simulink model "PVmppt"  (R2018b)
settings: Solver=FixedStepAuto  StartTime=0.0  StopTime=Inf  FixedStep=T  RelTol=1e-3
PostLoadFcn:
  | , if any(exist('dsrtsu_mdlpostloadfcn', 'file') ~= 0), dsrtsu_mdlpostloadfcn('Execute', bdroot); end,
InitFcn:
  | , if any(exist('dsmpb_private', 'file') ~= 0), dsmpb_private('dsmpb_mdlclblib', 'Init', bdroot); end,
values from neighbouring files (symbols this model uses):
  fixedgain_i1 = 10*1000/(3*100)    (= 33.3333333333)    [param.m]
  fixedgain_v3 = 10*22000/(3*100*2.5)    (= 293.333333333)    [param.m]
  fixedgain_v4 = 10*22000/(3*100*2.5)    (= 293.333333333)    [param.m]
  gain_i1 = 1    [param.m]
  gain_v1 = 1    [param.m]
  gain_v3 = 1    [param.m]
  gain_v4 = 1    [param.m]
  offset_i1 = 0.25    [param.m]
  offset_v1 = 0.15    [param.m]
  offset_v3 = 0.6    [param.m]
  offset_v4 = 0.2    [param.m]
undefined symbols (not defined in the file or in its folder): fixedgain_vc1
libraries: rti1202lib_adc_class1 x4, rtiproclib x3
PreSaveFcn:
  | , if any(exist('dsmpb_private', 'file') ~= 0), dsmpb_private('dsmpb_mdlclblib', 'PreSave', bdroot); end,
CloseFcn:
  | , if any(exist('dsmpb_private', 'file') ~= 0), dsmpb_private('dsmpb_mdlclblib', 'Close', bdroot); end,
Description:
  | Standard RTI1202 template.
  | Supported MATLAB version:  R2018b.
settings Model: Tag=RTI1202  DSRTSU_INTERNAL_RTI_VER=550  DSRTSU_INTERNAL_RTI_TYPE=rti1202  RTICANMMDATA=struct('GeneralSetupData',struct('modelroot','C:\marcos\LSPyC_Varios\BOOST','generalsettings',struct('filesettings',struct('destfolder',struct('Name','RTICANMM_FILES','Check',1),'buildfolder',struct('Name','.','Check',1),'AbsDestfolder',struct('Name','C:\marcos\LSPyC_Varios\BOOST\RTICANMM_FILES'),'AbsBuildfolder',struct('Name','C:\marcos\LSPyC_Varios\BOOST'))),'options',struct('addpaths',1,'rmpaths',1,'addtrcexclusion',true,'cannavigator',struct('checkmonitoring',0),'show_usrtrc',0,'use_usrtrc',0),'advanced',struct('options',ones(1,100)),'MPSetup',{{}},'RTI',struct('Type','RTI1202','Ver','7.13','Date','02-Nov-2019'),'modelname','PVmppt','block','PVmppt'))  DSRTSU_INTERNAL_RTIFPGA=150  DSMPB_ID_DATA={}  Creator=Admin  LastModifiedBy=Admin
settings OptimizationCC: BlockReduction=off  OptimizeBlockIOStorage=off  BufferReuse=off  GlobalBufferReuse=off  ExpressionFolding=off  LocalBlockOutputs=off  OptimizeDataStoreBuffers=off  BusAssignmentInplaceUpdate=off
settings DebuggingCC: LibraryContextMissingDiagnostic=none
settings HardwareCC: ProdBitPerPointer=32  ProdBitPerSizeT=32  ProdBitPerPtrDiffT=32  ProdLargestAtomicInteger=Integer  ProdEndianess=BigEndian  ProdWordSize=32  ProdHWDeviceType=Custom Processor->Custom  TargetIntDivRoundTo=Zero  TargetEndianess=BigEndian  TargetHWDeviceType=Custom Processor->Custom
settings SFSimCC: SimUseLocalCustomCode=off  MATLABDynamicMemAlloc=off
settings RTWCC: SystemTargetFile=rti1202.tlc  MakeCommand=make_rti  TemplateMakefile=rti1202.tmf  Description=dSPACE DS1202 Hardware Platform  RTWUseLocalCustomCode=off
settings CodeAppCC: StateflowObjectComments=on
settings STFCustomTargetCC: ParMdlRefBuildCompliant=on  SystemTargetFile=rti1202.tlc
settings GRTTargetCC: TargetLangStandard=C89/C90 (ANSI)  CompOptLevelCompliant=off  ConcurrentExecutionCompliant=off  CombineOutputUpdateFcns=off  MatFileLogging=off  CPPClassGenCompliant=off  UseToolchainInfoCompliant=off
settings ConfigComp: CovMetricSettings=dswe

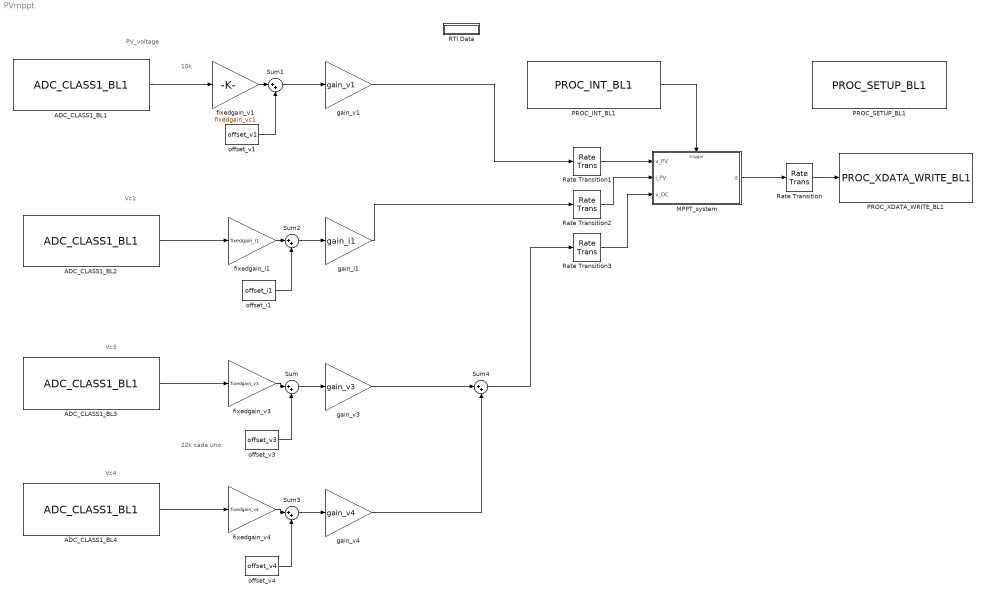
== system PVmppt ==
  note: 22k cada uno
  note: Vc3
  note: 10k
  note: Vc1
  note: PV_voltage
  note: Vc4
  ADC_CLASS1_BL1 : rti1202lib_adc_class1/ADC_CLASS1_BL1  DSProperties=struct('RTI',struct('Version',uint32(1),'BlockType',struct('isSLSource',uint8(1),'isSLSink',uint8(1),'isHWSource',uint8(0),'isHWSink',uint8(1),'isSetup',uint8(0),'isInline',uint8(1),'isNonInline',uint8(0),'isInterrupt',uint8(0),'isChannelwise',uint8(1)),'IOBoardType',{{'DS120X','STD','ADCC1'}},'UnitType','ADC','Identifier','ADC','DialogType','ML','BlockSet','NONE','SlaveProcessor','NONE'))  RTIBlockInterface=struct('InputPortsActive',0,'InputPortsWidth',int32(1),'InputPortsDataType',{{'SS_BOOLEAN'}},'InputPortsName',{{'Continue'}},'OutputPortsActive',[1 0],'OutputPortsWidth',int32([1 1]),'OutputPortsDataType',{{'SS_DOUBLE','SS_INT16'}},'OutputPortsName',{{'ADC','Status'}},'DialogFcn','rti120xstdadcc1adcgui','SampleTime',{{-1}},'InitLevel',3,'IconTransparency','on','BlockDisplay',{{['ADC CL1\nChannel: 1'],'center'}},'BlockName',struct('Token',{{'ADC_CLASS1_BL1'}}))  RTIBlockParameters=struct('ReadMode',{{1,'OFF',[1 2]}},'ChannelNo',{{1,'OFF',[]}},'ConversionMode',{{1,'OFF',[1 2]}},'TriggerSource',{{1,'OFF',[1 2]}},'TriggerLineIn',{{1,'OFF',[1 16]}},'SampleMode',{{1,'OFF',[1 2]}},'BurstTriggerSource',{{1,'OFF',[1 2]}},'BurstTriggerLine',{{1,'OFF',[1 16]}},'ConvTriggerSource',{{3,'OFF',[1 3]}},'ConvTriggerLine',{{1,'OFF',[1 16]}},'ConvPeriod',{{'100e-6','OFF',[1e-6 1.34]}},'ConvPeriodCheck',{{0,'OFF',[]}},'BurstSize',{{'10','OFF',[]}},'BurstSizeCheck',{{0,'OFF',[]}},'DataSetOffset',{{'0','OFF',[]}},'DataSetOffsetCheck',{{0,'OFF',[]}},'DataSetLength',{{'1','OFF',[]}},'DataSetLengthCheck',{{0,'OFF',[]}},'EnableTriggerEvent',{{0,'OFF',[0 1]}},'TriggerMode',{{2,'OFF',[1 3]}},'TriggerLineOut',{{1,'OFF',[1 16]}},'ADCSWStartEnable',{{0,'OFF',[0 1]}},'SampleTime',{{'-1','OFF',[-1 inf]}},'SampleTimeCheck',{{1,'OFF',[]}},'StatusPortEnable',{{0,'OFF',[0 1]}},'TLCFileName',{{'rti120xadc_c1_adc','OFF',[]}})  RTISFcnParameters=struct('ReadMode','int16','ChannelNo','int16','ConversionMode','int16','TriggerSource','int16','TriggerLineIn','int16','SampleMode','int16','BurstTriggerSource','int16','BurstTriggerLine','int16','ConvTriggerSource','int16','ConvTriggerLine','int16','ConvPeriod','double','BurstSize','int16','DataSetOffset','int16','DataSetLength','int16','EnableTriggerEvent','int16','TriggerMode','int16','TriggerLineOut','int16','ADCSWStartEnable','int16','SampleTime','double','StatusPortEnable','int16','TLCFileName','char')  RTIBlockParaDefault=struct('ReadMode',1,'ChannelNo',1,'ConversionMode',1,'TriggerSource',1,'TriggerLineIn',1,'SampleMode',1,'BurstTriggerSource',1,'BurstTriggerLine',1,'ConvTriggerSource',3,'ConvTriggerLine',1,'ConvPeriod',0.0001,'ConvPeriodCheck',0,'BurstSize',10,'BurstSizeCheck',0,'DataSetOffset',0,'DataSetOffsetCheck',0,'DataSetLength',1,'DataSetLengthCheck',0,'EnableTriggerEvent',0,'TriggerMode',2,'TriggerLineOut',1,'ADCSWStartEnable',0,'SampleTime',-1,'SampleTimeCheck',1,'StatusPortEnable',0,'TLCFileName','rti120xadc_c1_adc')
  ADC_CLASS1_BL2 : rti1202lib_adc_class1/ADC_CLASS1_BL1  DSProperties=struct('RTI',struct('Version',uint32(1),'BlockType',struct('isSLSource',uint8(1),'isSLSink',uint8(1),'isHWSource',uint8(0),'isHWSink',uint8(1),'isSetup',uint8(0),'isInline',uint8(1),'isNonInline',uint8(0),'isInterrupt',uint8(0),'isChannelwise',uint8(1)),'IOBoardType',{{'DS120X','STD','ADCC1'}},'UnitType','ADC','Identifier','ADC','DialogType','ML','BlockSet','NONE','SlaveProcessor','NONE'))  RTIBlockInterface=struct('InputPortsActive',0,'InputPortsWidth',int32(1),'InputPortsDataType',{{'SS_BOOLEAN'}},'InputPortsName',{{'Continue'}},'OutputPortsActive',[1 0],'OutputPortsWidth',int32([1 1]),'OutputPortsDataType',{{'SS_DOUBLE','SS_INT16'}},'OutputPortsName',{{'ADC','Status'}},'DialogFcn','rti120xstdadcc1adcgui','SampleTime',{{-1}},'InitLevel',3,'IconTransparency','on','BlockDisplay',{{['ADC CL1\nChannel: 9'],'center'}},'BlockName',struct('Token',{{'ADC_CLASS1_BL1'}}))  RTIBlockParameters=struct('ReadMode',{{1,'OFF',[1 2]}},'ChannelNo',{{9,'OFF',[]}},'ConversionMode',{{1,'OFF',[1 2]}},'TriggerSource',{{1,'OFF',[1 2]}},'TriggerLineIn',{{1,'OFF',[1 16]}},'SampleMode',{{1,'OFF',[1 2]}},'BurstTriggerSource',{{1,'OFF',[1 2]}},'BurstTriggerLine',{{1,'OFF',[1 16]}},'ConvTriggerSource',{{3,'OFF',[1 3]}},'ConvTriggerLine',{{1,'OFF',[1 16]}},'ConvPeriod',{{'100e-6','OFF',[1e-6 1.34]}},'ConvPeriodCheck',{{0,'OFF',[]}},'BurstSize',{{'10','OFF',[]}},'BurstSizeCheck',{{0,'OFF',[]}},'DataSetOffset',{{'0','OFF',[]}},'DataSetOffsetCheck',{{0,'OFF',[]}},'DataSetLength',{{'1','OFF',[]}},'DataSetLengthCheck',{{0,'OFF',[]}},'EnableTriggerEvent',{{0,'OFF',[0 1]}},'TriggerMode',{{2,'OFF',[1 3]}},'TriggerLineOut',{{1,'OFF',[1 16]}},'ADCSWStartEnable',{{0,'OFF',[0 1]}},'SampleTime',{{'-1','OFF',[-1 inf]}},'SampleTimeCheck',{{1,'OFF',[]}},'StatusPortEnable',{{0,'OFF',[0 1]}},'TLCFileName',{{'rti120xadc_c1_adc','OFF',[]}})  RTISFcnParameters=struct('ReadMode','int16','ChannelNo','int16','ConversionMode','int16','TriggerSource','int16','TriggerLineIn','int16','SampleMode','int16','BurstTriggerSource','int16','BurstTriggerLine','int16','ConvTriggerSource','int16','ConvTriggerLine','int16','ConvPeriod','double','BurstSize','int16','DataSetOffset','int16','DataSetLength','int16','EnableTriggerEvent','int16','TriggerMode','int16','TriggerLineOut','int16','ADCSWStartEnable','int16','SampleTime','double','StatusPortEnable','int16','TLCFileName','char')  RTIBlockParaDefault=struct('ReadMode',1,'ChannelNo',1,'ConversionMode',1,'TriggerSource',1,'TriggerLineIn',1,'SampleMode',1,'BurstTriggerSource',1,'BurstTriggerLine',1,'ConvTriggerSource',3,'ConvTriggerLine',1,'ConvPeriod',0.0001,'ConvPeriodCheck',0,'BurstSize',10,'BurstSizeCheck',0,'DataSetOffset',0,'DataSetOffsetCheck',0,'DataSetLength',1,'DataSetLengthCheck',0,'EnableTriggerEvent',0,'TriggerMode',2,'TriggerLineOut',1,'ADCSWStartEnable',0,'SampleTime',-1,'SampleTimeCheck',1,'StatusPortEnable',0,'TLCFileName','rti120xadc_c1_adc')
  ADC_CLASS1_BL3 : rti1202lib_adc_class1/ADC_CLASS1_BL1  DSProperties=struct('RTI',struct('Version',uint32(1),'BlockType',struct('isSLSource',uint8(1),'isSLSink',uint8(1),'isHWSource',uint8(0),'isHWSink',uint8(1),'isSetup',uint8(0),'isInline',uint8(1),'isNonInline',uint8(0),'isInterrupt',uint8(0),'isChannelwise',uint8(1)),'IOBoardType',{{'DS120X','STD','ADCC1'}},'UnitType','ADC','Identifier','ADC','DialogType','ML','BlockSet','NONE','SlaveProcessor','NONE'))  RTIBlockInterface=struct('InputPortsActive',0,'InputPortsWidth',int32(1),'InputPortsDataType',{{'SS_BOOLEAN'}},'InputPortsName',{{'Continue'}},'OutputPortsActive',[1 0],'OutputPortsWidth',int32([1 1]),'OutputPortsDataType',{{'SS_DOUBLE','SS_INT16'}},'OutputPortsName',{{'ADC','Status'}},'DialogFcn','rti120xstdadcc1adcgui','SampleTime',{{-1}},'InitLevel',3,'IconTransparency','on','BlockDisplay',{{['ADC CL1\nChannel: 3'],'center'}},'BlockName',struct('Token',{{'ADC_CLASS1_BL1'}}))  RTIBlockParameters=struct('ReadMode',{{1,'OFF',[1 2]}},'ChannelNo',{{3,'OFF',[]}},'ConversionMode',{{1,'OFF',[1 2]}},'TriggerSource',{{1,'OFF',[1 2]}},'TriggerLineIn',{{1,'OFF',[1 16]}},'SampleMode',{{1,'OFF',[1 2]}},'BurstTriggerSource',{{1,'OFF',[1 2]}},'BurstTriggerLine',{{1,'OFF',[1 16]}},'ConvTriggerSource',{{3,'OFF',[1 3]}},'ConvTriggerLine',{{1,'OFF',[1 16]}},'ConvPeriod',{{'100e-6','OFF',[1e-6 1.34]}},'ConvPeriodCheck',{{0,'OFF',[]}},'BurstSize',{{'10','OFF',[]}},'BurstSizeCheck',{{0,'OFF',[]}},'DataSetOffset',{{'0','OFF',[]}},'DataSetOffsetCheck',{{0,'OFF',[]}},'DataSetLength',{{'1','OFF',[]}},'DataSetLengthCheck',{{0,'OFF',[]}},'EnableTriggerEvent',{{0,'OFF',[0 1]}},'TriggerMode',{{2,'OFF',[1 3]}},'TriggerLineOut',{{1,'OFF',[1 16]}},'ADCSWStartEnable',{{0,'OFF',[0 1]}},'SampleTime',{{'-1','OFF',[-1 inf]}},'SampleTimeCheck',{{1,'OFF',[]}},'StatusPortEnable',{{0,'OFF',[0 1]}},'TLCFileName',{{'rti120xadc_c1_adc','OFF',[]}})  RTISFcnParameters=struct('ReadMode','int16','ChannelNo','int16','ConversionMode','int16','TriggerSource','int16','TriggerLineIn','int16','SampleMode','int16','BurstTriggerSource','int16','BurstTriggerLine','int16','ConvTriggerSource','int16','ConvTriggerLine','int16','ConvPeriod','double','BurstSize','int16','DataSetOffset','int16','DataSetLength','int16','EnableTriggerEvent','int16','TriggerMode','int16','TriggerLineOut','int16','ADCSWStartEnable','int16','SampleTime','double','StatusPortEnable','int16','TLCFileName','char')  RTIBlockParaDefault=struct('ReadMode',1,'ChannelNo',1,'ConversionMode',1,'TriggerSource',1,'TriggerLineIn',1,'SampleMode',1,'BurstTriggerSource',1,'BurstTriggerLine',1,'ConvTriggerSource',3,'ConvTriggerLine',1,'ConvPeriod',0.0001,'ConvPeriodCheck',0,'BurstSize',10,'BurstSizeCheck',0,'DataSetOffset',0,'DataSetOffsetCheck',0,'DataSetLength',1,'DataSetLengthCheck',0,'EnableTriggerEvent',0,'TriggerMode',2,'TriggerLineOut',1,'ADCSWStartEnable',0,'SampleTime',-1,'SampleTimeCheck',1,'StatusPortEnable',0,'TLCFileName','rti120xadc_c1_adc')
  ADC_CLASS1_BL4 : rti1202lib_adc_class1/ADC_CLASS1_BL1  DSProperties=struct('RTI',struct('Version',uint32(1),'BlockType',struct('isSLSource',uint8(1),'isSLSink',uint8(1),'isHWSource',uint8(0),'isHWSink',uint8(1),'isSetup',uint8(0),'isInline',uint8(1),'isNonInline',uint8(0),'isInterrupt',uint8(0),'isChannelwise',uint8(1)),'IOBoardType',{{'DS120X','STD','ADCC1'}},'UnitType','ADC','Identifier','ADC','DialogType','ML','BlockSet','NONE','SlaveProcessor','NONE'))  RTIBlockInterface=struct('InputPortsActive',0,'InputPortsWidth',int32(1),'InputPortsDataType',{{'SS_BOOLEAN'}},'InputPortsName',{{'Continue'}},'OutputPortsActive',[1 0],'OutputPortsWidth',int32([1 1]),'OutputPortsDataType',{{'SS_DOUBLE','SS_INT16'}},'OutputPortsName',{{'ADC','Status'}},'DialogFcn','rti120xstdadcc1adcgui','SampleTime',{{-1}},'InitLevel',3,'IconTransparency','on','BlockDisplay',{{['ADC CL1\nChannel: 4'],'center'}},'BlockName',struct('Token',{{'ADC_CLASS1_BL1'}}))  RTIBlockParameters=struct('ReadMode',{{1,'OFF',[1 2]}},'ChannelNo',{{4,'OFF',[]}},'ConversionMode',{{1,'OFF',[1 2]}},'TriggerSource',{{1,'OFF',[1 2]}},'TriggerLineIn',{{1,'OFF',[1 16]}},'SampleMode',{{1,'OFF',[1 2]}},'BurstTriggerSource',{{1,'OFF',[1 2]}},'BurstTriggerLine',{{1,'OFF',[1 16]}},'ConvTriggerSource',{{3,'OFF',[1 3]}},'ConvTriggerLine',{{1,'OFF',[1 16]}},'ConvPeriod',{{'100e-6','OFF',[1e-6 1.34]}},'ConvPeriodCheck',{{0,'OFF',[]}},'BurstSize',{{'10','OFF',[]}},'BurstSizeCheck',{{0,'OFF',[]}},'DataSetOffset',{{'0','OFF',[]}},'DataSetOffsetCheck',{{0,'OFF',[]}},'DataSetLength',{{'1','OFF',[]}},'DataSetLengthCheck',{{0,'OFF',[]}},'EnableTriggerEvent',{{0,'OFF',[0 1]}},'TriggerMode',{{2,'OFF',[1 3]}},'TriggerLineOut',{{1,'OFF',[1 16]}},'ADCSWStartEnable',{{0,'OFF',[0 1]}},'SampleTime',{{'-1','OFF',[-1 inf]}},'SampleTimeCheck',{{1,'OFF',[]}},'StatusPortEnable',{{0,'OFF',[0 1]}},'TLCFileName',{{'rti120xadc_c1_adc','OFF',[]}})  RTISFcnParameters=struct('ReadMode','int16','ChannelNo','int16','ConversionMode','int16','TriggerSource','int16','TriggerLineIn','int16','SampleMode','int16','BurstTriggerSource','int16','BurstTriggerLine','int16','ConvTriggerSource','int16','ConvTriggerLine','int16','ConvPeriod','double','BurstSize','int16','DataSetOffset','int16','DataSetLength','int16','EnableTriggerEvent','int16','TriggerMode','int16','TriggerLineOut','int16','ADCSWStartEnable','int16','SampleTime','double','StatusPortEnable','int16','TLCFileName','char')  RTIBlockParaDefault=struct('ReadMode',1,'ChannelNo',1,'ConversionMode',1,'TriggerSource',1,'TriggerLineIn',1,'SampleMode',1,'BurstTriggerSource',1,'BurstTriggerLine',1,'ConvTriggerSource',3,'ConvTriggerLine',1,'ConvPeriod',0.0001,'ConvPeriodCheck',0,'BurstSize',10,'BurstSizeCheck',0,'DataSetOffset',0,'DataSetOffsetCheck',0,'DataSetLength',1,'DataSetLengthCheck',0,'EnableTriggerEvent',0,'TriggerMode',2,'TriggerLineOut',1,'ADCSWStartEnable',0,'SampleTime',-1,'SampleTimeCheck',1,'StatusPortEnable',0,'TLCFileName','rti120xadc_c1_adc')
  MPPT_system : Subsystem
  PROC_INT_BL1 : rtiproclib/PROC_INT_BL1  DSProperties=struct('RTI',struct('Version',uint32(4),'BlockType',struct('isSLSource',uint8(1),'isSLSink',uint8(0),'isHWSource',uint8(0),'isHWSink',uint8(0),'isSetup',uint8(1),'isInline',uint8(1),'isNonInline',uint8(0),'isInterrupt',uint8(0),'isChannelwise',uint8(0)),'IOBoardType','DSPROC','UnitType','','Identifier','INT','DialogType','ML','BlockSet','DSPROC','SlaveProcessor',''))  RTIBlockInterface=struct('OutputPortsActive',1,'OutputPortsWidth',int32(1),'OutputPortsName',{{'Interrupt'}},'FunctionCall',uint32(0),'DialogFcn','rtiprocintgui','InitLevel',3,'BlockDisplay',{{['Interrupt In 1\nintPV \nBoard: 1'],'center'}},'IconTransparency','on','BlockName',struct('Token',{{'PROC_INT_BL1'}}))  RTIBlockParameters=struct('BoardNo',{{'1','OFF',[1 16]}},'ChannelNo',{{'1','OFF',[1 8]}},'AccessTyp',{{'Interrupt','OFF',[]}},'BinaryPoint',{{'0','OFF',[]}},'DataFormat',{{'unsigned','OFF',[]}},'BufferLength',{{'0','OFF',[]}},'MultiChAccess',{{'0','OFF',[]}},'ModelPortBlock',{{{struct('BlockId','9610b641-06eb-474b-93d9-1fe1a2450546','SignalId','67497c73-3a4b-49d7-9d73-6a8e13bb9408')},'OFF',[]}})  RTISFcnParameters=struct('BoardNo','double','ChannelNo','double','AccessTyp','char','BinaryPoint','double','DataFormat','char','BufferLength','double')  RTIBlockParaDefault=struct('BoardNo','1','ChannelNo','1','AccessTyp','Interrupt','BinaryPoint','10','DataFormat','unsigned','BufferLength','0','MultiChAccess','0','ModelPortBlock',{{struct('BlockId','','SignalId','')}})
  PROC_SETUP_BL1 : rtiproclib/PROC_SETUP_BL1  DSProperties=struct('RTI',struct('Version',uint32(3),'BlockType',struct('isSLSource',uint8(0),'isSLSink',uint8(0),'isHWSource',uint8(0),'isHWSink',uint8(0),'isSetup',uint8(1),'isInline',uint8(1),'isNonInline',uint8(0),'isInterrupt',uint8(0),'isChannelwise',uint8(0)),'IOBoardType','DSPROC','UnitType','SETUP','Identifier','SETUP','DialogType','ML','BlockSet','NONE','SlaveProcessor',''))  RTIBlockInterface=struct('OutputPortsWidth',int32(0),'OutputPortsActive',0,'InitLevel',3,'DialogFcn','rtiprocsetupgui','BlockDisplay',{{['Processor Setup'],'auto'}},'IconTransparency','off','BlockName',struct('Token',{{'PROC_SETUP_BL1'}}))  RTIBlockParameters=struct('NumBoardsUsed',{{1,'OFF',[1 16]}},'ModelMode',{{2,'OFF',[]}},'IniFileList',{{struct('Fullname','','Filename','','Relname','','Assigned',0),'OFF',[]}},'SubsysList',{{struct('SharedAccess',1,'SetupBlockHandle',165.000244140625,'SetupBlockName','FPGA_SETUP_BL1','SubsysName','FPGA','SubsysHandle',9.000244140625,'SubsysPath','/FPGA','Assigned',1,'IniFilePath','C:\marcos\LSPyC_Varios\BOOST\PVmppt_rtiFPGA/INI/FPGA_81ECA2A96C331B.ini','IniFileName','FPGA_81ECA2A96C331B','IniFileDate',739856.6984722222),'OFF',[]}},'AssignList',{{struct('BoardNumber',{1,2,3,4,5,6,7,8,9,10,11,12,13,14,15,16},'ModelType',{1,0,0,0,0,0,0,0,0,0,0,0,0,0,0,0},'ModelNo',{1,0,0,0,0,0,0,0,0,0,0,0,0,0,0,0},'ProgOption',{2,0,0,0,0,0,0,0,0,0,0,0,0,0,0,0},'IncludeBuild',{1,0,0,0,0,0,0,0,0,0,0,0,0,0,0,0},'IncludeProcAppl',{true,0,0,0,0,0,0,0,0,0,0,0,0,0,0,0}),'OFF',[]}},'ProcSetupHandles',{{-1,'OFF',[]}},'MaxNumBoards',{{16,'OFF',[]}},'ModelPath',{{'C:\marcos\LSPyC_Varios\BOOST','OFF',[]}},'FrameDir',{{[' '],'OFF',[]}},'TLCFileName',{{'rtiprocsetup','OFF',[]}},'IsNewBlock',{{0,'OFF',[]}},'NeedsCodeGen',{{0,'OFF',[]}})  RTISFcnParameters=struct('FrameDir','char','TLCFileName','char')  RTIBlockParaDefault=struct('NumBoardsUsed',1,'ModelMode',1,'IniFileList',struct('Fullname','','Filename','','Relname','','Assigned',''),'SubsysList',struct('SubsysName','','SubsysPath','','SubsysHandle','','SetupBlockHandle','','SetupBlockName','','Filename','','Relname','','IniFilePath','','IniFileName','','IniFileDate','','Assigned',''),'AssignList',struct('BoardNumber','','ModelType','','ModelNo','','ProgOption','','IncludeBuild','','IncludeProcAppl',''),'ProcSetupHandles',-1,'MaxNumBoards',16,'ModelPath',[' '],'FrameDir',[' '],'TLCFileName','rtiprocsetup','IsNewBlock',1,'NeedsCodeGen',0)
      settings: AttributesFormatString=Processor-Build
  PROC_XDATA_WRITE_BL1 : rtiproclib/PROC_XDATA_WRITE_BL1  DSProperties=struct('RTI',struct('Version',uint32(5),'BlockType',struct('isSLSource',uint8(0),'isSLSink',uint8(1),'isHWSource',uint8(0),'isHWSink',uint8(0),'isSetup',uint8(0),'isInline',uint8(1),'isNonInline',uint8(0),'isInterrupt',uint8(0),'isChannelwise',uint8(0)),'IOBoardType','DSPROC','UnitType','','Identifier','PHSWRITE','DialogType','ML','BlockSet','DSPROC','SlaveProcessor',''))  RTIBlockInterface=struct('InputPortsActive',true,'InputPortsWidth',{{'DYNAMICALLY_SIZED'}},'InputPortsDataType',{{'SS_DOUBLE'}},'InputPortsName',{{'Data'}},'InitLevel',3,'DialogFcn','rtiprocphswritegui','BlockDisplay',{{['Register Out 1\ndPV \nGroup: 1 Board: 1'],'auto'}},'IconTransparency','on','BlockName',struct('Token',{{'PROC_XDATA_WRITE_BL1'}}))  RTIBlockParameters=struct('BoardNo',{{'1','OFF',[1 16]}},'ChannelNo',{{'1','OFF',[]}},'AccessTyp',{{'Register','OFF',[]}},'BinaryPoint',{{'0','OFF',[]}},'DataFormat',{{'signed','OFF',[]}},'BufferLength',{{'0','OFF',[]}},'GroupNo',{{'1','OFF',[]}},'MultiChAccess',{{'0','OFF',[]}},'InitOnly',{{'0','OFF',[]}},'InitValue',{{'0','OFF',[]}},'TLCFileName',{{'rtiprocphswrite','OFF',[]}},'ModelPortBlock',{{{struct('BlockId','2f1dfd25-acce-472a-9be8-beaf3aa11d6f','SignalId','30c39a49-0e5b-4009-83ab-185a20087ab0','SignalPath',{{'data'}})},'OFF',[]}})  RTISFcnParameters=struct('BoardNo','double','ChannelNo','double','GroupNo','double','AccessTyp','char','BinaryPoint','double','DataFormat','char','BufferLength','double','InitOnly','double','InitValue','double','TLCFileName','char')  RTIBlockParaDefault=struct('BoardNo','1','ChannelNo','0','AccessTyp','Register','BinaryPoint','10','DataFormat','signed','BufferLength','16','GroupNo','0','MultiChAccess','0','InitOnly','0','InitValue','0','TLCFileName','rtiprocphswrite','ModelPortBlock',{{struct('BlockId','','SignalId','','BusObject','')}})
  RTI Data : Subsystem  Tag=struct('RTIDataServer',struct('RTIDataServerVs','2','RTIModelDescription','struct(''main'',''PVmppt'',''sub'','''',''isMp'',0)'))  LoadFcn="if exist('rtidc'), try,  rtidc('DataHostBlockClbLoad', gcbh); catch, disp(['Warning: ''LoadFcn'' for RTI Data block failed: ' lasterr]); end, end,"  mask(RTI_DATA_HOST){}
      mask help:
      | RTI Data Block.
      | This block is used by RTI to store internal model-dependent data.
      | Please keep this block on the root level of the model. Deleting this block will result in data loss.
      |
      | NEVER DELETE OR COPY THIS BLOCK!
      settings: CopyFcn="if exist('rtidc'), try,  rtidc('DataHostBlockClbCopy', gcbh); catch, disp(['Warning: ''CopyFcn'' for RTI Data block failed: ' lasterr]); end, end,"  DeleteFcn="if exist('rtidc'), try,  rtidc('DataHostBlockClbDelete', gcbh); catch, disp(['Warning: ''DeleteFcn'' for RTI Data block failed: ' lasterr]); end, end,"  ModelCloseFcn="if exist('rtidc'), try,  rtidc('DataHostBlockClbModelClose', gcbh); catch, disp(['Warning: ''ModelCloseFcn'' for RTI Data block failed: ' lasterr]); end, end,"  PreSaveFcn="if exist('rtidc'), try,  rtidc('DataHostBlockClbPreSave', gcbh); catch, disp(['Warning: ''PreSaveFcn'' for RTI Data block failed: ' lasterr]); end, end,"  PostSaveFcn="if exist('rtidc'), try,  rtidc('DataHostBlockClbPostSave', gcbh); catch, disp(['Warning: ''PostSaveFcn'' for RTI Data block failed: ' lasterr]); end, end,"  NameChangeFcn="if exist('rtidc'), try,  rtidc('DataHostBlockClbNameChange', gcbh); catch, disp(['Warning: ''NameChangeFcn'' for RTI Data block failed: ' lasterr]); end, end,"
      mask Help:
      | RTI Data Block.
      | This block is used by RTI to store internal model-dependent data.
      | Please keep this block on the root level of the model. Deleting this block will result in data loss.
      | 
      | NEVER DELETE OR COPY THIS BLOCK!
      mask Display:
      | text(0.5, 0.5, 'RTI Data', 'HorizontalAlignment', 'center');
      | plot([1 0]);
  Rate Transition{,1..3} (4 alike) : RateTransition  Deterministic=off  OutPortSampleTimeOpt=Inherit
  Sum{,1..4} (5 alike) : Sum  Inputs=|++
  fixedgain_i1 : Gain  Gain=fixedgain_i1
  fixedgain_v1 : Gain  Gain=fixedgain_vc1
  fixedgain_v3 : Gain  Gain=fixedgain_v3
  fixedgain_v4 : Gain  Gain=fixedgain_v4
  gain_i1 : Gain  Gain=gain_i1
  gain_v1 : Gain  Gain=gain_v1
  gain_v3 : Gain  Gain=gain_v3
  gain_v4 : Gain  Gain=gain_v4
  offset_i1 : Constant  Value=offset_i1
  offset_v1 : Constant  Value=offset_v1
  offset_v3 : Constant  Value=offset_v3
  offset_v4 : Constant  Value=offset_v4
  wires:
  ADC_CLASS1_BL2/1 -> fixedgain_i1/1
  ADC_CLASS1_BL1/1 -> fixedgain_v1/1
  gain_i1/1 -> Rate Transition2/1
  gain_v3/1 -> Sum4/1
  ADC_CLASS1_BL3/1 -> fixedgain_v3/1
  Rate Transition2/1 -> MPPT_system/2(i_PV)
  Rate Transition1/1 -> MPPT_system/1(v_PV)
  offset_v3/1 -> Sum/2
  offset_v1/1 -> Sum1/2
  Rate Transition3/1 -> MPPT_system/3(v_DC)
  gain_v1/1 -> Rate Transition1/1
  Sum2/1 -> gain_i1/1
  fixedgain_i1/1 -> Sum2/1
  fixedgain_v1/1 -> Sum1/1
  Sum/1 -> gain_v3/1
  Sum1/1 -> gain_v1/1
  MPPT_system/1(d) -> Rate Transition/1
  offset_i1/1 -> Sum2/2
  fixedgain_v3/1 -> Sum/1
  PROC_INT_BL1/1 -> MPPT_system/Trigger
  Rate Transition/1 -> PROC_XDATA_WRITE_BL1/1
  Sum3/1 -> gain_v4/1
  offset_v4/1 -> Sum3/2
  fixedgain_v4/1 -> Sum3/1
  gain_v4/1 -> Sum4/2
  ADC_CLASS1_BL4/1 -> fixedgain_v4/1
  Sum4/1 -> Rate Transition3/1

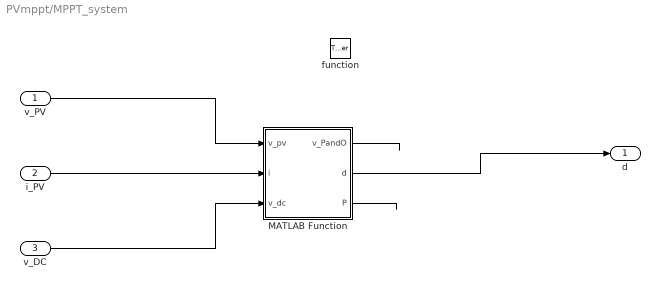
== system PVmppt/MPPT_system ==
  v_PV : Inport
  i_PV : Inport  Port=2
  v_DC : Inport  Port=3
  function : TriggerPort  TriggerType=function-call  VariantControl=Variant
  MATLAB Function : MATLAB Function  TreatAsAtomicUnit=on
  d : Outport  VectorParamsAs1DForOutWhenUnconnected=on
  wires:
  MATLAB Function/2(d) -> d/1
  i_PV/1 -> MATLAB Function/2(i)
  MATLAB Function/1(v_PandO) -> ?
  v_PV/1 -> MATLAB Function/1(v_pv)
  v_DC/1 -> MATLAB Function/3(v_dc)
  MATLAB Function/3(P) -> ?

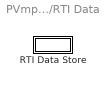
== system PVmppt/RTI Data ==
  RTI Data Store : Subsystem  Tag="struct('private',struct('version',struct('dsVer',uint32(2),'dsVerCreation',uint32(2),'RTI',struct('ver','7.13','type','RTI1202')),'access',struct('type','Model','isPerm',1,'created',['22-Aug-2025 16:30:34'],'modified',['28-Aug-2025 16:29:05'],'location','')),'public',struct('main',struct('data',[]),'sub',struct('name',{{'PVmppt'}},'data',{{struct('TH',struct('thTaskInfo',struct('taskType',{'TIMER','HWINT','TMRINT','SWINT','GLINT'},'tasksNumOf',{1,1,0,0,0},'srcIds',{{'TIMERA'},{'FPGACL1FPGA_INTP0Ch0'},{},{},{}},'taskNames',{{['Timer Task 1']},{'PROC_INT_BL1'},{},{},{}})),'th_tc',struct('dataType',{'TASK','TASK'},'taskGroupId',{'',''},'taskGroupList',{{},{}},'taskSchedulingPolicy',{'FCFS','FCFS'},'taskType',{'TIMER','HWINT'},'blkh',{-1,['PVmppt/PROC_INT_BL1/Common Hardware' char(10) 'Interrupt Interface']},'srcId',{'TIMERA','FPGACL1FPGA_INTP0Ch0'},'srcSgnName',{['Timer A interrupt'],['FPGA Type CL1 FPGA_INT Port 0 Channel 0']},'srcCpuName',{'',''},'taskName',{['Timer Task 1  [5e-05] s'],'PROC_INT_BL1'},'taskNameDisplayExt',{'',''},'smplTime',{5e-5,0},'smplTimeOffs',{0,0},'hasFixedPriority',{0,0},'priority',{1,2},'hasFixedOvc',{0,0},'ovcType',{1,1},'ovcMax',{1,1}),'tc_th',struct('dataType',{'TASK','TASK'},'taskGroupId',{'',''},'taskGroupList',{{},{}},'taskSchedulingPolicy',{'FCFS','FCFS'},'taskType',{'TIMER','HWINT'},'blkh',{-1,['PVmppt/PROC_INT_BL1/Common Hardware' char(10) 'Interrupt Interface']},'srcId',{'TIMERA','FPGACL1FPGA_INTP0Ch0'},'srcSgnName',{['Timer A interrupt'],['FPGA Type CL1 FPGA_INT Port 0 Channel 0']},'srcCpuName',{'',''},'taskName',{['Timer Task 1  [5e-05] s'],'PROC_INT_BL1'},'taskNameDisplayExt',{'',''},'smplTime',{5e-5,0},'smplTimeOffs',{0,0},'hasFixedPriority',{0,0},'priority',{1,2},'hasFixedOvc',{0,0},'ovcType',{1,1},'ovcMax',{1,1}))}})))"  mask(RTI_DATA_STORE){}
      mask help:
      | RTI Data Store Block. This block is used by RTI to store internal model dependent data. Deleting this block will result in data loss.
      |
      | NEVER DELETE, COPY, OR MODIFY THIS BLOCK!
      mask Help:
      | RTI Data Store Block. This block is used by RTI to store internal model dependent data. Deleting this block will result in data loss.
      | 
      | NEVER DELETE, COPY, OR MODIFY THIS BLOCK!
      mask Display: text(0.5, 0.5, ' ', 'HorizontalAlignment', 'center');

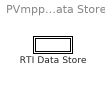
== system PVmppt/RTI Data/RTI Data Store ==
  RTI Data Store : Subsystem  mask(RTI_DATA_STORE){}
      mask help:
      | RTI Data Store Block. This block is used by RTI to store internal model dependent data. Deleting this block will result in data loss.
      |
      | NEVER DELETE, COPY, OR MODIFY THIS BLOCK!
      mask Help:
      | RTI Data Store Block. This block is used by RTI to store internal model dependent data. Deleting this block will result in data loss.
      | 
      | NEVER DELETE, COPY, OR MODIFY THIS BLOCK!
      mask Display: text(0.5, 0.5, ' ', 'HorizontalAlignment', 'center');

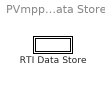
== system PVmppt/RTI Data/RTI Data Store/RTI Data Store ==
  RTI Data Store : Subsystem  mask(RTI_DATA_STORE){}
      mask help:
      | RTI Data Store Block. This block is used by RTI to store internal model dependent data. Deleting this block will result in data loss.
      |
      | NEVER DELETE, COPY, OR MODIFY THIS BLOCK!
      mask Help:
      | RTI Data Store Block. This block is used by RTI to store internal model dependent data. Deleting this block will result in data loss.
      | 
      | NEVER DELETE, COPY, OR MODIFY THIS BLOCK!
      mask Display: text(0.5, 0.5, ' ', 'HorizontalAlignment', 'center');

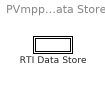
== system PVmppt/RTI Data/RTI Data Store/RTI Data Store/RTI Data Store ==
  RTI Data Store : Subsystem  mask(RTI_DATA_STORE){}
      mask help:
      | RTI Data Store Block. This block is used by RTI to store internal model dependent data. Deleting this block will result in data loss.
      |
      | NEVER DELETE, COPY, OR MODIFY THIS BLOCK!
      mask Help:
      | RTI Data Store Block. This block is used by RTI to store internal model dependent data. Deleting this block will result in data loss.
      | 
      | NEVER DELETE, COPY, OR MODIFY THIS BLOCK!
      mask Display: text(0.5, 0.5, ' ', 'HorizontalAlignment', 'center');

== system PVmppt/RTI Data/RTI Data Store/RTI Data Store/RTI Data Store/RTI Data Store ==

== matlab function PVmppt/MPPT_system/MATLAB Function ==
  data: v_pv input; v_PandO output; i input; v_dc input; d output; P output
function [v_PandO, d, P] = MPPT(v_pv,i, v_dc)
persistent P_ant v_ref v_ant v_dc_ant

if isempty(P_ant)
    P_ant = 0;
    v_ref = 10;
    v_ant = 10;
end


P = v_pv*i;

v_dc_ant = v_dc;
delta = P-P_ant;

if (abs(delta) < 0.001)
elseif delta > 0
        if v_pv>v_ant
            v_ref = v_ref+.1;
        else
            v_ref = v_ref-.1;
        end
else
        if v_pv>v_ant
            v_ref = v_ref-.1;
        else
            v_ref = v_ref+.1;
        end
end
if v_ref>15
    v_ref = 15;
end
if v_ref<0
    v_ref = 0;
end
P_ant = P;
v_ant = v_pv;

v_PandO = v_ref;


g = v_dc_ant/v_ref;
d = 100*(1-(1/g)); %debe coincidir con el PWM de la FPGA (no el de interrupcion)
if d<2
    d = 2;
elseif d>98
    d=98;
end
